simulink library "commanapbnd2"  (Simulink 6.0)
undefined symbols (not defined in the file or in its folder): den, num
libraries: dspsigattribs x26, commanapbnd2 x2, commblksprivate x2, commsynccomp2 x2, dspsrcs4 x1
settings Model: RequirementInfo=9  CovMetricSettings=d  Creator=tdelve  LastModifiedBy=ysong  ExtModeAutoUpdateStatusClock=off

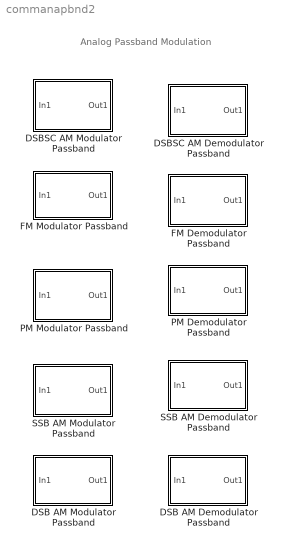
== system commanapbnd2 ==
  note: Analog Passband Modulation
  DSB AM Demodulator Passband : Subsystem  mask(DSB AM Demodulator Passband){Offset=1, Fc=100, Ph=0, num=[4.57 9.14 4.57]*.01, den=[1 -1.3108 .4936], ts=0.001}
      mask prompts: Offset "Offset factor:"; Fc "Carrier frequency (Hz):"; Ph "Initial phase (rad):"; num "Lowpass filter numerator:"; den "Lowpass filter denominator:"; ts "Sample time (s):"
      mask help: Demodulate a double-sideband amplitude modulated signal. The input signal must be a sample-based scalar. The output is a 1-D scalar.
      mask init:
      | if ((length(Ph)~=1) | (length(Offset)~=1) | (length(ts)~=1) | (length(Fc)~=1))error('Mask parameters must be scalar values.');end;
      mask Help: helpview(commbhelp)
      mask Display:
      | plot(0,0,100,100,[5+4.5*[0:.15:10] 50 50 50 50+4.5*[0:10]],[85+10*[sin([0:.15:10]*pi*2+cumsum(sin([0:.15:10]*pi/5))/2)] 85 99 75   10*sin([0:10]*pi/5)+85]);
      | disp('DSB AM')
  DSB AM Modulator Passband : Subsystem  mask(DSB AM Modulator Passband){Offset=1, Fc=100, Ph=0}
      mask prompts: Offset "Input signal offset:"; Fc "Carrier frequency (Hz):"; Ph "Initial phase (rad):"
      mask help: Modulate the input signal using the double-sideband amplitude modulation method. The input signal must be a sample-based scalar. The output is a 1-D scalar.
      mask init:
      | if ((length(Ph)~=1) | (length(Fc)~=1) | (length(Offset)~=1))error('Mask parameters must be scalar values.');end;
      mask Help: helpview(commbhelp)
      mask Display:
      | plot(0,0,100,100,[4.5*[0:10]+5 50 50 50 50+4.5*[0:.15:10]],[10*sin([0:10]*pi/5)+85 85 99 75 85+10*[sin([0:.15:10]*pi*2+cumsum(sin([0:.15:10]*pi/5))/2)]]);
      | disp('DSB AM')
  DSBSC AM Demodulator Passband : Subsystem  mask(DSBSC AM Demodulator Passband){Fc=100, num=[4.57 9.14 4.57]*.01, den=[1 -1.3108 .4936], Ph=pi/2, ts=0.001}
      mask prompts: Fc "Carrier frequency (Hz):"; num "Lowpass filter numerator:"; den "Lowpass filter denominator:"; Ph "Initial phase (rad):"; ts "Sample time (s):"
      mask help: Demodulate a double-sideband suppressed carrier amplitude modulated signal. The input signal must be a sample-based scalar. The output is a 1-D scalar.
      mask init:
      | if ((length(Ph)~=1) | (length(Fc)~=1) | (length(ts)~=1))error('Mask parameters must be scalar values.');end;
      | pi2=pi*2;
      mask Help: helpview(commbhelp)
      mask Display:
      | plot(0,0,100,100,[5+4.5*[0:.15:10] 50 50 50 50+4.5*[0:10]],[85+10*[sin([0:.15:10]*pi*2+cumsum(sin([0:.15:10]*pi/5))/2)] 85 99 75   10*sin([0:10]*pi/5)+85]);
      | disp('DSBSC AM')
  DSBSC AM Modulator Passband : Subsystem  mask(DSBSC AM Modulator Passband){Fc=100, Ph=pi/2}
      mask prompts: Fc "Carrier frequency (Hz):"; Ph "Initial phase (rad):"
      mask help: Modulate the input signal using the double-sideband suppressed carrier amplitude modulation method. The input signal must be a sample-based scalar. The output is a 1-D scalar.
      mask init:
      | if ((length(Ph)~=1) | (length(Fc)~=1))error('Mask parameters must be scalar values.');end;
      | Fc=Fc*2*pi;
      mask Help: helpview(commbhelp)
      mask Display:
      | plot(0,0,100,100,[4.5*[0:10]+5 50 50 50 50+4.5*[0:.15:10]],[10*sin([0:10]*pi/5)+85 85 99 75 85+10*[sin([0:.15:10]*pi*2+cumsum(sin([0:.15:10]*pi/5))/2)]]);
      | disp('DSBSC AM')
  FM Demodulator Passband : Subsystem  mask(FM Demodulator Passband){Fc=100, Ph=0, HzPerVolt=1, num=[4.57 9.14 4.57]*.01, den=[1 -1.3108 .4936], ts=0.001}
      mask prompts: Fc "Carrier frequency (Hz):"; Ph "Initial phase (rad):"; HzPerVolt "Modulation constant (Hertz per volt):"; num "Lowpass filter numerator:"; den "Lowpass filter denominator:"; ts "Sample time (s):"
      mask help: Demodulate a frequency modulated signal using a phase-locked loop. The input signal must be a sample-based scalar. The output is a 1-D scalar.
      mask init:
      | if ((length(Ph)~=1) | (length(HzPerVolt)~=1) | (length(ts)~=1) | (length(Fc)~=1))error('Mask parameters must be scalar values.');end;
      | Ph=Ph+pi/2;
      mask Help: helpview(commbhelp)
      mask Display:
      | plot(0,0,100,100,[5+4.5*[0:.15:10] 50 50 50 50+4.5*[0:10]],[85+10*[sin([0:.15:10]*pi*2+cumsum(sin([0:.15:10]*pi/5))/2)] 85 99 75   10*sin([0:10]*pi/5)+85]);
      | disp('FM')
  FM Modulator Passband : Subsystem  mask(FM Modulator Passband){Fc=100, Ph=0, HzPerV=1, ts=0.001, td=Inf}
      mask prompts: Fc "Carrier frequency (Hz):"; Ph "Initial phase (rad):"; HzPerV "Modulation constant (Hertz per volt):"; ts "Sample time (s):"; td "Symbol interval (s, Use Inf for analog mod);"
      mask help: Modulate the input signal using the frequency modulation method. The input signal must be a sample-based scalar. The output is a 1-D scalar.
      mask init:
      | if ((length(Ph)~=1) | (length(HzPerV)~=1) | (length(ts)~=1) | (length(td)~=1) | (length(Fc)~=1))error('Mask parameters must be scalar values.');end;
      | Kc=HzPerV;pi2=2*pi;if isinf(td),td=realmax;end;
      mask Help: helpview(commbhelp)
      mask Display:
      | plot(0,0,100,100,[4.5*[0:10]+5 50 50 50 50+4.5*[0:.15:10]],[10*sin([0:10]*pi/5)+85 85 99 75 85+10*[sin([0:.15:10]*pi*2+cumsum(sin([0:.15:10]*pi/5))/2)]]);
      | disp('FM')
  PM Demodulator Passband : Subsystem  mask(PM Demodulator Passband){Fc=100, Ph=0, Kc=1, num=[4.57 9.14 4.57]*.01, den=[1 -1.3108 .4936], HzPerVolt=1, ts=0.001}
      mask prompts: Fc "Carrier frequency (Hz):"; Ph "Initial phase (rad):"; Kc "Modulation constant (Radians per volt):"; num "Lowpass filter numerator:"; den "Lowpass filter denominator:"; HzPerVolt "VCO Gain (Hertz per volt):"; ts "Sample time (s):"
      mask help: Demodulate a phase modulated signal using a phase-locked loop. The input signal must be a sample-based scalar. The output is a 1-D scalar.
      mask init:
      | Ph=Ph+pi/2;
      | Kv=2*pi*HzPerVolt;
      mask Help: helpview(commbhelp)
      mask Display:
      | plot(0,0,100,100,[5+4.5*[0:.15:10] 50 50 50 50+4.5*[0:10]],[85+10*[sin([0:.15:10]*pi*2+cumsum(sin([0:.15:10]*pi/5))/2)] 85 99 75   10*sin([0:10]*pi/5)+85]);
      | disp('PM')
  PM Modulator Passband : Subsystem  mask(PM Modulator Passband){Fc=100, Ph=0, Kc=1, td=Inf}
      mask prompts: Fc "Carrier frequency (Hz):"; Ph "Initial phase (rad):"; Kc "Modulation constant (Radians per volt):"; td "Symbol interval (s, Use inf for analog case):"
      mask help: Modulate the input signal using the phase modulation method. The input signal must be a sample-based scalar. The output is a 1-D scalar.
      mask init:
      | if ((length(Ph)~=1) | (length(Kc)~=1) | (length(td)~=1) | (length(Fc)~=1))error('Mask parameters must be scalar values.');end;
      | Fc=Fc*2*pi;if isinf(td),td=realmax;end;
      mask Help: helpview(commbhelp)
      mask Display:
      | plot(0,0,100,100,[4.5*[0:10]+5 50 50 50 50+4.5*[0:.15:10]],[10*sin([0:10]*pi/5)+85 85 99 75 85+10*[sin([0:.15:10]*pi*2+cumsum(sin([0:.15:10]*pi/5))/2)]]);
      | disp('PM')
  SSB AM Demodulator Passband : Subsystem  mask(SSB AM Demodulator Passband){Fc=100, num=[4.57 9.14 4.57]*.01, den=[1 -1.3108 .4936], Ph=0, ts=0.001}
      mask prompts: Fc "Carrier frequency (Hz):"; num "Lowpass filter numerator:"; den "Lowpass filter denominator:"; Ph "Initial phase (rad):"; ts "Sample time (s):"
      mask help: Demodulate a single-sideband amplitude modulated signal. The input signal must be a sample-based scalar. The output is a 1-D scalar.
      mask init:
      | if ((length(Ph)~=1) | (length(Fc)~=1) | (length(ts)~=1))error('Mask parameters must be scalar values.');end;
      | Fc=Fc*2*pi;Pg=Ph+pi/2;
      mask Help: helpview(commbhelp)
      mask Display:
      | plot(0,0,100,100,[5+4.5*[0:.15:10] 50 50 50 50+4.5*[0:10]],[85+10*[sin([0:.15:10]*pi*2+cumsum(sin([0:.15:10]*pi/5))/2)] 85 99 75   10*sin([0:10]*pi/5)+85]);
      | disp('SSB AM')
  SSB AM Modulator Passband : Subsystem  mask(SSB AM Modulator Passband){Fc=100, Ph=0, ban=10, dly=0.01, ts=0.001, sd=upper}
      mask prompts: Fc "Carrier frequency (Hz):"; Ph "Initial phase (rad):"; ban "Bandwidth of the input signal (Hz):"; dly "Time delay for Hilbert transform filter (s):"; ts "Sample time (s):"; sd "Sideband to modulate:"
      mask help: Modulate the input signal using the single-sideband amplitude modulation method with Hilbert transform filter. The input signal must be a sample-based scalar. The output is a 1-D scalar.
      mask init:
      | if ((length(Ph)~=1) | (length(ban)~=1) | (length(ts)~=1) | (length(dly)~=1) | (length(Fc)~=1))error('Mask parameters must be scalar values.');end;
      | if dly/ts<3 error('Time delay is too small compared to the Sample time value');end;
      | if ban>1/ts, ban=1/ts-ts;end;
      | if(dly/ts>1000)
      | error(['The filter coefficients will take too long to compute.'...
      |         'Try reducing the length of the impulse response by increasing the sample time, or decreasing the delay'])
      | else
      | [num,den]=hilbiir(ts,dly,ban);pi2=2*pi;pih=pi/2;
      | k=-1;if lower(sd)=='lower',k=1;end;
      | end;
      mask Help: helpview(commbhelp)
      mask StyleString: edit,edit,edit,edit,edit,popup(Upper|Lower)
      mask Display:
      | plot(0,0,100,100,[4.5*[0:10]+5 50 50 50 50+4.5*[0:.15:10]],[10*sin([0:10]*pi/5)+85 85 99 75 85+10*[sin([0:.15:10]*pi*2+cumsum(sin([0:.15:10]*pi/5))/2)]]);
      | disp('SSB AM')

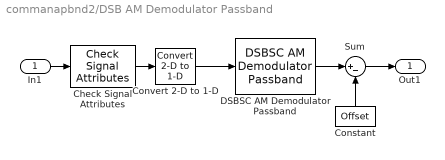
== system commanapbnd2/DSB AM Demodulator Passband ==
  In1 : Inport
  Check Signal Attributes : dspsigattribs/Check Signal Attributes  SigAttribCheckMethod=Does not match attributes exactly  Complexity=Ignore  Frame=Sample-based  DimsCheckMethod=Is...  Dimensions=Scalar (1-D or 2-D)  DatatypeCheckMethod=Ignore  DatatypeGeneral=Boolean  DtypeFloatSpecific=Any floating-point  DtypeFixedSpecific=Any fixed-point  DtypeIntSpecific=Any integer  SampleMode=Ignore
  Constant : Constant  Orientation=up  Value=Offset
  Convert 2-D to 1-D : dspsigattribs/Convert 2-D to 1-D
  DSBSC AM Demodulator Passband : commanapbnd2/DSBSC AM Demodulator Passband  Fc=Fc  num=num  den=den  Ph=Ph  ts=ts
  Sum : Sum  Inputs=|+-  SaturateOnIntegerOverflow=on  InputSameDT=on
  Out1 : Outport
  wires:
  Constant/1 -> Sum/2
  DSBSC AM Demodulator Passband/1 -> Sum/1
  In1/1 -> Check Signal Attributes/1
  Sum/1 -> Out1/1
  Convert 2-D to 1-D/1 -> DSBSC AM Demodulator Passband/1
  Check Signal Attributes/1 -> Convert 2-D to 1-D/1

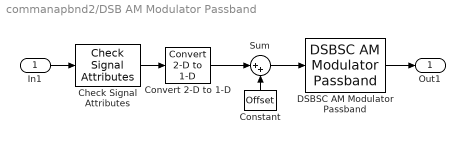
== system commanapbnd2/DSB AM Modulator Passband ==
  In1 : Inport
  Check Signal Attributes : dspsigattribs/Check Signal Attributes  SigAttribCheckMethod=Does not match attributes exactly  Complexity=Ignore  Frame=Sample-based  DimsCheckMethod=Is...  Dimensions=Scalar (1-D or 2-D)  DatatypeCheckMethod=Ignore  DatatypeGeneral=Boolean  DtypeFloatSpecific=Any floating-point  DtypeFixedSpecific=Any fixed-point  DtypeIntSpecific=Any integer  SampleMode=Ignore
  Constant : Constant  Orientation=up  Value=Offset
  Convert 2-D to 1-D : dspsigattribs/Convert 2-D to 1-D
  DSBSC AM Modulator Passband : commanapbnd2/DSBSC AM Modulator Passband  Fc=Fc  Ph=Ph
  Sum : Sum  Inputs=|++  SaturateOnIntegerOverflow=on  InputSameDT=on
  Out1 : Outport
  wires:
  Constant/1 -> Sum/2
  Sum/1 -> DSBSC AM Modulator Passband/1
  In1/1 -> Check Signal Attributes/1
  DSBSC AM Modulator Passband/1 -> Out1/1
  Convert 2-D to 1-D/1 -> Sum/1
  Check Signal Attributes/1 -> Convert 2-D to 1-D/1

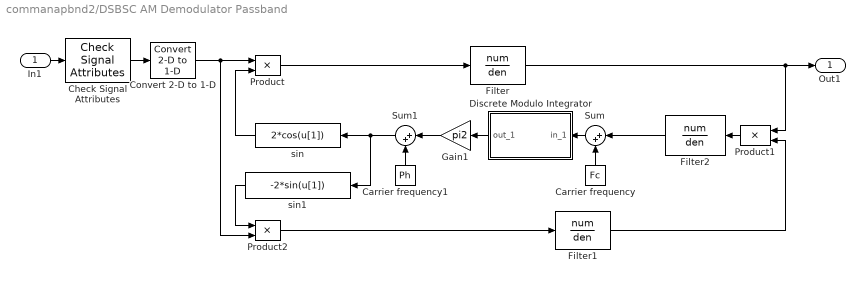
== system commanapbnd2/DSBSC AM Demodulator Passband ==
  In1 : Inport
  Carrier frequency : Constant  Orientation=up  Value=Fc
  Carrier frequency1 : Constant  Orientation=up  Value=Ph
  Check Signal Attributes : dspsigattribs/Check Signal Attributes  SigAttribCheckMethod=Does not match attributes exactly  Complexity=Ignore  Frame=Sample-based  DimsCheckMethod=Is...  Dimensions=Scalar (1-D or 2-D)  DatatypeCheckMethod=Ignore  DatatypeGeneral=Boolean  DtypeFloatSpecific=Any floating-point  DtypeFixedSpecific=Any fixed-point  DtypeIntSpecific=Any integer  SampleMode=Ignore
  Convert 2-D to 1-D : dspsigattribs/Convert 2-D to 1-D
  Discrete Modulo Integrator : Subsystem  Orientation=left  mask(Discrete Modulo Integrator){method=Forward Euler, modu=1, init=0, ts=ts}
      mask prompts: method "Integration method:"; modu "Absolute value bound:"; init "Initial condition:"; ts "Sample time:"
      mask help:
      | Integrate the input signal in discrete time and then uses the Absolute value bound parameter, K, to produce output strictly between -K and K. The block uses the rem function in MATLAB.
      |
      | The input can be either a scalar, a sample-based vector, or a frame-based row vector.  This block processes each vector element independently.
      mask init:
      | commblkdmodint(gcb);
      settings: ErrorFcn=commblkdmint
      mask Help: helpview(commbhelp)
      mask StyleString: popup(Forward Euler|Backward Euler|Trapezoidal),edit,edit,edit
      mask Display: disp('Discrete\nModulo\nIntegrator')
  Filter : DiscreteFilter  Numerator=num  Denominator=den  SampleTime=ts
  Filter1 : DiscreteFilter  Numerator=num  Denominator=den  SampleTime=ts
  Filter2 : DiscreteFilter  Orientation=left  Numerator=num  Denominator=den  SampleTime=ts
  Gain1 : Gain  Orientation=left  Gain=pi2  SaturateOnIntegerOverflow=on
  Product : Product  SaturateOnIntegerOverflow=on  InputSameDT=on
  Product1 : Product  Orientation=left  SaturateOnIntegerOverflow=on  InputSameDT=on
  Product2 : Product  SaturateOnIntegerOverflow=on  InputSameDT=on
  Sum : Sum  Orientation=left  Inputs=|++  SaturateOnIntegerOverflow=on  InputSameDT=on
  Sum1 : Sum  Orientation=left  Inputs=|++  SaturateOnIntegerOverflow=on  InputSameDT=on
  sin : Fcn  Orientation=left  Expr=2*cos(u[1])
  sin1 : Fcn  Orientation=left  Expr=-2*sin(u[1])
  Out1 : Outport
  wires:
  Sum1/1 -> sin/1, sin1/1
  Filter2/1 -> Sum/1
  Product/1 -> Filter/1
  sin/1 -> Product/2
  Carrier frequency/1 -> Sum/2
  Sum/1 -> Discrete Modulo Integrator/1(in_1)
  Product1/1 -> Filter2/1
  sin1/1 -> Product2/1
  In1/1 -> Check Signal Attributes/1
  Product2/1 -> Filter1/1
  Filter1/1 -> Product1/2
  Discrete Modulo Integrator/1(out_1) -> Gain1/1
  Gain1/1 -> Sum1/1
  Carrier frequency1/1 -> Sum1/2
  Filter/1 -> Product1/1, Out1/1
  Convert 2-D to 1-D/1 -> Product/1, Product2/2
  Check Signal Attributes/1 -> Convert 2-D to 1-D/1

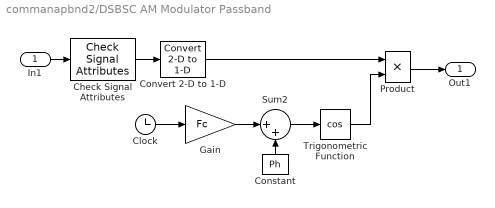
== system commanapbnd2/DSBSC AM Modulator Passband ==
  In1 : Inport
  Check Signal Attributes : dspsigattribs/Check Signal Attributes  SigAttribCheckMethod=Does not match attributes exactly  Complexity=Ignore  Frame=Sample-based  DimsCheckMethod=Is...  Dimensions=Scalar (1-D or 2-D)  DatatypeCheckMethod=Ignore  DatatypeGeneral=Boolean  DtypeFloatSpecific=Any floating-point  DtypeFixedSpecific=Any fixed-point  DtypeIntSpecific=Any integer  SampleMode=Ignore
  Clock : Clock
      settings: Decimation=10
  Constant : Constant  Orientation=up  Value=Ph
  Convert 2-D to 1-D : dspsigattribs/Convert 2-D to 1-D
  Gain : Gain  Gain=Fc  SaturateOnIntegerOverflow=on
  Product : Product  SaturateOnIntegerOverflow=on  InputSameDT=on
  Sum2 : Sum  Inputs=|++  SaturateOnIntegerOverflow=on  InputSameDT=on
  Trigonometric Function : Trigonometry  Operator=cos
  Out1 : Outport
  wires:
  Trigonometric Function/1 -> Product/2
  In1/1 -> Check Signal Attributes/1
  Clock/1 -> Gain/1
  Gain/1 -> Sum2/1
  Constant/1 -> Sum2/2
  Sum2/1 -> Trigonometric Function/1
  Product/1 -> Out1/1
  Convert 2-D to 1-D/1 -> Product/1
  Check Signal Attributes/1 -> Convert 2-D to 1-D/1

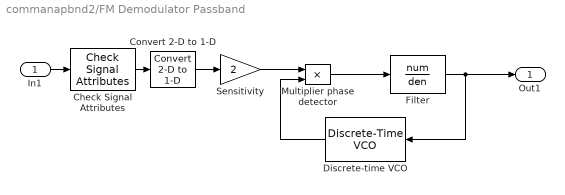
== system commanapbnd2/FM Demodulator Passband ==
  In1 : Inport
  Check Signal Attributes : dspsigattribs/Check Signal Attributes  SigAttribCheckMethod=Does not match attributes exactly  Complexity=Ignore  Frame=Sample-based  DimsCheckMethod=Is...  Dimensions=Scalar (1-D or 2-D)  DatatypeCheckMethod=Ignore  DatatypeGeneral=Boolean  DtypeFloatSpecific=Any floating-point  DtypeFixedSpecific=Any fixed-point  DtypeIntSpecific=Any integer  SampleMode=Ignore
  Convert 2-D to 1-D : dspsigattribs/Convert 2-D to 1-D
  Discrete-time VCO : commsynccomp2/Discrete-Time VCO  Orientation=left  Ac=1  Fc=Fc  Kc=HzPerVolt  Ph=Ph  ts=ts
  Filter : DiscreteFilter  Numerator=num  Denominator=den  SampleTime=ts
  Multiplier phase detector : Product  SaturateOnIntegerOverflow=on  InputSameDT=on
  Sensitivity : Gain  Gain=2  SaturateOnIntegerOverflow=on
  Out1 : Outport
  wires:
  Discrete-time VCO/1 -> Multiplier phase detector/2
  Multiplier phase detector/1 -> Filter/1
  Filter/1 -> Discrete-time VCO/1, Out1/1
  In1/1 -> Check Signal Attributes/1
  Sensitivity/1 -> Multiplier phase detector/1
  Convert 2-D to 1-D/1 -> Sensitivity/1
  Check Signal Attributes/1 -> Convert 2-D to 1-D/1

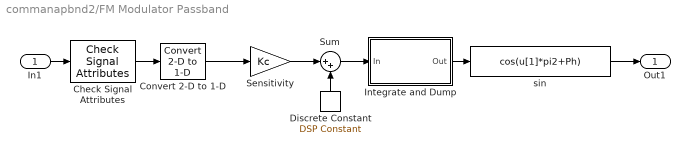
== system commanapbnd2/FM Modulator Passband ==
  In1 : Inport
  Check Signal Attributes : dspsigattribs/Check Signal Attributes  SigAttribCheckMethod=Does not match attributes exactly  Complexity=Ignore  Frame=Sample-based  DimsCheckMethod=Is...  Dimensions=Scalar (1-D or 2-D)  DatatypeCheckMethod=Ignore  DatatypeGeneral=Boolean  DtypeFloatSpecific=Any floating-point  DtypeFixedSpecific=Any fixed-point  DtypeIntSpecific=Any integer  SampleMode=Ignore
  Convert 2-D to 1-D : dspsigattribs/Convert 2-D to 1-D
  Discrete Constant : dspsrcs4/DSP Constant  Orientation=up  Value=Fc  SampleMode=Discrete  discreteOutput=Sample-based (interpret vectors as 1-D)  continuousOutput=Sample-based  sampTime=ts  framePeriod=ts  dataType=Inherit from 'Constant value'  wordLen=16  udDataType=sfix(16)  fracBitsMode=Best precision  numFracBits=15  InterpretAs1D=on  Ts=ts  FramebasedOutput=off
  Integrate and Dump : Subsystem  mask(Integrate and Dump){limit=Inf/2, td=td, ts=ts}
      mask prompts: limit "Absolute value bound:"; td "Integration period (s):"; ts "Sample time:"
      mask help:
      | Integrate the input signal in discrete time over the Integration period and then reduce modulo the Absolute value bound parameter. The integrator resets its internal state before integrating the next period.
      |
      | The input can be either a scalar, a sample-based vector, or a frame-based row vector.  This block processes each vector element independently.
      mask init:
      | limit(find(isinf(limit))) = realmax;
      | td(find(isinf(td))) = realmax;
      | 
      | if(~isempty(ts))
      |    if(length(ts) ~= 1)
      |       error('Sample time parameter must be a real scalar.');
      |    end;
      | end;
      settings: ErrorFcn=commblkintdmp
      mask Help: helpview(commbhelp)
      mask Display: disp('Integrate\nand Dump')
  Sensitivity : Gain  Gain=Kc  SaturateOnIntegerOverflow=on
  Sum : Sum  Inputs=|++  SaturateOnIntegerOverflow=on  InputSameDT=on
  sin : Fcn  Expr=cos(u[1]*pi2+Ph)
  Out1 : Outport
  wires:
  Integrate and Dump/1(Out) -> sin/1
  Sum/1 -> Integrate and Dump/1(In)
  In1/1 -> Check Signal Attributes/1
  Sensitivity/1 -> Sum/1
  sin/1 -> Out1/1
  Convert 2-D to 1-D/1 -> Sensitivity/1
  Check Signal Attributes/1 -> Convert 2-D to 1-D/1
  Discrete Constant/1 -> Sum/2

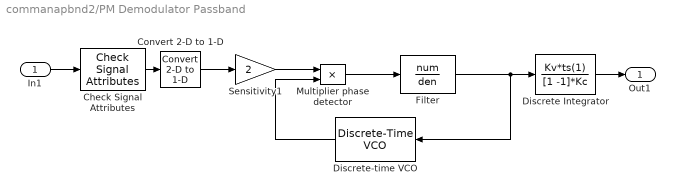
== system commanapbnd2/PM Demodulator Passband ==
  In1 : Inport
  Check Signal Attributes : dspsigattribs/Check Signal Attributes  SigAttribCheckMethod=Does not match attributes exactly  Complexity=Ignore  Frame=Sample-based  DimsCheckMethod=Is...  Dimensions=Scalar (1-D or 2-D)  DatatypeCheckMethod=Ignore  DatatypeGeneral=Boolean  DtypeFloatSpecific=Any floating-point  DtypeFixedSpecific=Any fixed-point  DtypeIntSpecific=Any integer  SampleMode=Ignore
  Convert 2-D to 1-D : dspsigattribs/Convert 2-D to 1-D
  Discrete Integrator : DiscreteFilter  Numerator=Kv*ts(1)  Denominator=[1 -1]*Kc  SampleTime=ts
  Discrete-time VCO : commsynccomp2/Discrete-Time VCO  Orientation=left  Ac=1  Fc=Fc  Kc=HzPerVolt  Ph=Ph  ts=ts
  Filter : DiscreteFilter  Numerator=num  Denominator=den  SampleTime=ts
  Multiplier phase detector : Product  SaturateOnIntegerOverflow=on  InputSameDT=on
  Sensitivity1 : Gain  Gain=2  SaturateOnIntegerOverflow=on
  Out1 : Outport  InitialOutput=0
  wires:
  Discrete-time VCO/1 -> Multiplier phase detector/2
  Filter/1 -> Discrete-time VCO/1, Discrete Integrator/1
  Multiplier phase detector/1 -> Filter/1
  In1/1 -> Check Signal Attributes/1
  Sensitivity1/1 -> Multiplier phase detector/1
  Discrete Integrator/1 -> Out1/1
  Convert 2-D to 1-D/1 -> Sensitivity1/1
  Check Signal Attributes/1 -> Convert 2-D to 1-D/1

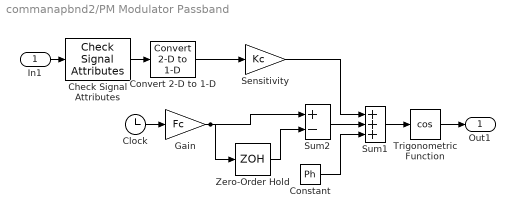
== system commanapbnd2/PM Modulator Passband ==
  In1 : Inport
  Check Signal Attributes : dspsigattribs/Check Signal Attributes  SigAttribCheckMethod=Does not match attributes exactly  Complexity=Ignore  Frame=Sample-based  DimsCheckMethod=Is...  Dimensions=Scalar (1-D or 2-D)  DatatypeCheckMethod=Ignore  DatatypeGeneral=Boolean  DtypeFloatSpecific=Any floating-point  DtypeFixedSpecific=Any fixed-point  DtypeIntSpecific=Any integer  SampleMode=Ignore
  Clock : Clock
      settings: Decimation=10
  Constant : Constant  Value=Ph
  Convert 2-D to 1-D : dspsigattribs/Convert 2-D to 1-D
  Gain : Gain  Gain=Fc  SaturateOnIntegerOverflow=on
  Sensitivity : Gain  Gain=Kc  SaturateOnIntegerOverflow=on
  Sum1 : Sum  Inputs=+++  SaturateOnIntegerOverflow=on  InputSameDT=on
  Sum2 : Sum  Inputs=+-  SaturateOnIntegerOverflow=on  InputSameDT=on
  Trigonometric Function : Trigonometry  Operator=cos
  Zero-Order Hold : ZeroOrderHold  SampleTime=td
  Out1 : Outport
  wires:
  Constant/1 -> Sum1/3
  Sum1/1 -> Trigonometric Function/1
  Clock/1 -> Gain/1
  Sum2/1 -> Sum1/2
  Zero-Order Hold/1 -> Sum2/2
  Gain/1 -> Sum2/1, Zero-Order Hold/1
  In1/1 -> Check Signal Attributes/1
  Sensitivity/1 -> Sum1/1
  Trigonometric Function/1 -> Out1/1
  Convert 2-D to 1-D/1 -> Sensitivity/1
  Check Signal Attributes/1 -> Convert 2-D to 1-D/1

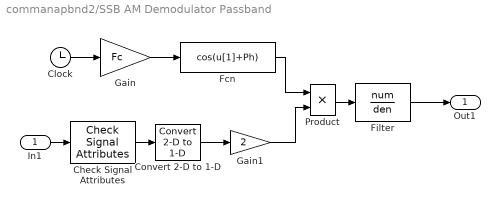
== system commanapbnd2/SSB AM Demodulator Passband ==
  In1 : Inport
  Check Signal Attributes : dspsigattribs/Check Signal Attributes  SigAttribCheckMethod=Does not match attributes exactly  Complexity=Ignore  Frame=Sample-based  DimsCheckMethod=Is...  Dimensions=Scalar (1-D or 2-D)  DatatypeCheckMethod=Ignore  DatatypeGeneral=Boolean  DtypeFloatSpecific=Any floating-point  DtypeFixedSpecific=Any fixed-point  DtypeIntSpecific=Any integer  SampleMode=Ignore
  Clock : Clock
      settings: Decimation=10
  Convert 2-D to 1-D : dspsigattribs/Convert 2-D to 1-D
  Fcn : Fcn  Expr=cos(u[1]+Ph)
  Filter : DiscreteFilter  Numerator=num  Denominator=den  SampleTime=ts
  Gain : Gain  Gain=Fc  SaturateOnIntegerOverflow=on
  Gain1 : Gain  Gain=2  SaturateOnIntegerOverflow=on
  Product : Product  SaturateOnIntegerOverflow=on  InputSameDT=on
  Out1 : Outport
  wires:
  Clock/1 -> Gain/1
  Product/1 -> Filter/1
  Fcn/1 -> Product/1
  Gain1/1 -> Product/2
  Gain/1 -> Fcn/1
  Filter/1 -> Out1/1
  Convert 2-D to 1-D/1 -> Gain1/1
  Check Signal Attributes/1 -> Convert 2-D to 1-D/1
  In1/1 -> Check Signal Attributes/1

== system commanapbnd2/SSB AM Modulator Passband ==
  In1 : Inport
  Check Signal Attributes : dspsigattribs/Check Signal Attributes  SigAttribCheckMethod=Does not match attributes exactly  Complexity=Ignore  Frame=Sample-based  DimsCheckMethod=Is...  Dimensions=Scalar (1-D or 2-D)  DatatypeCheckMethod=Ignore  DatatypeGeneral=Boolean  DtypeFloatSpecific=Any floating-point  DtypeFixedSpecific=Any fixed-point  DtypeIntSpecific=Any integer  SampleMode=Ignore
  Convert 2-D to 1-D : dspsigattribs/Convert 2-D to 1-D
  Filter : DiscreteFilter  Numerator=num  Denominator=den  SampleTime=ts
  Gain : Gain  Gain=k  SaturateOnIntegerOverflow=on
  QAM passband : Subsystem  mask(QAM Passband){Fc=Fc, Ph=Ph}
      mask prompts: Fc "Carrier frequency (Hz):"; Ph "Initial phase (rad):"
      mask help: Modulate the in-phase signal from first input port and quadrature signal from the second port using QAM.
      mask init:
      | Fc=Fc*2*pi;
      mask Help: helpview(commbhelp)
      mask Display:
      | plot(0,0,100,100,[4.5*[0:10]+5 50 50 50 50+4.5*[0:.3:10]],[10*sin([0:10]*pi/5)+85 85 99 75 85+10*[sin([0:.3:10]*pi/5).*sin([0:.3:10]*pi*2)]]);
      | disp('\nPassband\nQAM')
  Out1 : Outport
  wires:
  In1/1 -> Check Signal Attributes/1
  Filter/1 -> Gain/1
  Gain/1 -> QAM passband/2(in_2)
  QAM passband/1(out_1) -> Out1/1
  Convert 2-D to 1-D/1 -> QAM passband/1(in_1), Filter/1
  Check Signal Attributes/1 -> Convert 2-D to 1-D/1

== system commanapbnd2/DSBSC AM Demodulator Passband/Discrete Modulo Integrator ==
  in_1 : Inport
  Discrete Modulo Integrator : Subsystem
  "Exclude Frame-based Input " : dspsigattribs/Check Signal Attributes  SigAttribCheckMethod=Matches attributes exactly  Complexity=Ignore  Frame=Frame-based  DimsCheckMethod=Is not...  Dimensions=Row vector (2-D) or scalar  DatatypeCheckMethod=Ignore  DatatypeGeneral=Boolean  DtypeFloatSpecific=Any floating-point  DtypeFixedSpecific=Any fixed-point  DtypeIntSpecific=Any integer  SampleMode=Ignore
  Exclude Full Matrix : dspsigattribs/Check Signal Attributes  SigAttribCheckMethod=Matches attributes exactly  Complexity=Ignore  Frame=Ignore  DimsCheckMethod=Is...  Dimensions=Full matrix (2-D)  DatatypeCheckMethod=Ignore  DatatypeGeneral=Boolean  DtypeFloatSpecific=Any floating-point  DtypeFixedSpecific=Any fixed-point  DtypeIntSpecific=Any integer  SampleMode=Ignore
  Frame Status Conversion : dspsigattribs/Frame Status Conversion  growRefPort=off  outframe=Sample-based
  Inherit Shape : commblksprivate/Inherit Shape
  out_1 : Outport  InitialOutput=0
  wires:
  Discrete Modulo Integrator/1(Out1) -> Inherit Shape/1
  Frame Status Conversion/1 -> Discrete Modulo Integrator/1(In1)
  "Exclude Frame-based Input "/1 -> Frame Status Conversion/1
  Exclude Full Matrix/1 -> "Exclude Frame-based Input "/1
  Inherit Shape/1 -> out_1/1
  in_1/1 -> Inherit Shape/2, Exclude Full Matrix/1

== system commanapbnd2/FM Modulator Passband/Integrate and Dump ==
  In : Inport
  "Exclude Frame-based Input " : dspsigattribs/Check Signal Attributes  SigAttribCheckMethod=Matches attributes exactly  Complexity=Ignore  Frame=Frame-based  DimsCheckMethod=Is not...  Dimensions=Row vector (2-D) or scalar  DatatypeCheckMethod=Ignore  DatatypeGeneral=Boolean  DtypeFloatSpecific=Any floating-point  DtypeFixedSpecific=Any fixed-point  DtypeIntSpecific=Any integer  SampleMode=Ignore
  Exclude Full Matrix : dspsigattribs/Check Signal Attributes  SigAttribCheckMethod=Matches attributes exactly  Complexity=Ignore  Frame=Ignore  DimsCheckMethod=Is...  Dimensions=Full matrix (2-D)  DatatypeCheckMethod=Ignore  DatatypeGeneral=Boolean  DtypeFloatSpecific=Any floating-point  DtypeFixedSpecific=Any fixed-point  DtypeIntSpecific=Any integer  SampleMode=Ignore
  Frame Status Conversion : dspsigattribs/Frame Status Conversion  growRefPort=off  outframe=Sample-based
  Inherit Shape : commblksprivate/Inherit Shape
  Scheduled reset-int : S-Function  FunctionName=schdint  Parameters=td, ts, limit
  Out : Outport  InitialOutput=0
  wires:
  Exclude Full Matrix/1 -> "Exclude Frame-based Input "/1
  "Exclude Frame-based Input "/1 -> Frame Status Conversion/1
  Frame Status Conversion/1 -> Scheduled reset-int/1
  Inherit Shape/1 -> Out/1
  Scheduled reset-int/1 -> Inherit Shape/1
  In/1 -> Inherit Shape/2, Exclude Full Matrix/1

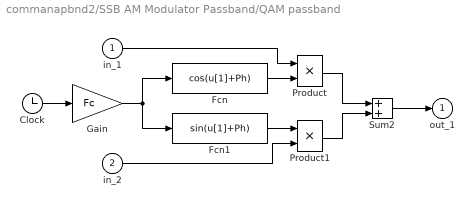
== system commanapbnd2/SSB AM Modulator Passband/QAM passband ==
  in_1 : Inport
  in_2 : Inport  Port=2
  Clock : Clock
      settings: Decimation=10
  Fcn : Fcn  Expr=cos(u[1]+Ph)
  Fcn1 : Fcn  Expr=sin(u[1]+Ph)
  Gain : Gain  Gain=Fc  SaturateOnIntegerOverflow=on
  Product : Product  SaturateOnIntegerOverflow=on  InputSameDT=on
  Product1 : Product  SaturateOnIntegerOverflow=on  InputSameDT=on
  Sum2 : Sum  SaturateOnIntegerOverflow=on  InputSameDT=on
  out_1 : Outport  InitialOutput=0
  wires:
  Sum2/1 -> out_1/1
  Fcn/1 -> Product/2
  in_1/1 -> Product/1
  Fcn1/1 -> Product1/1
  in_2/1 -> Product1/2
  Product/1 -> Sum2/1
  Product1/1 -> Sum2/2
  Clock/1 -> Gain/1
  Gain/1 -> Fcn1/1, Fcn/1

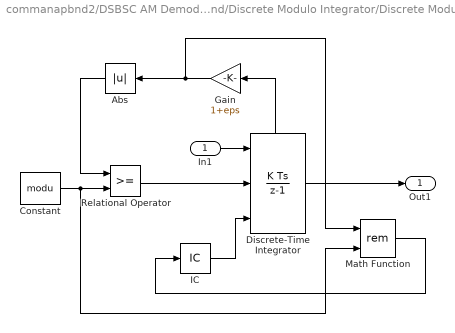
== system commanapbnd2/DSBSC AM Demodulator Passband/Discrete Modulo Integrator/Discrete Modulo Integrator ==
  In1 : Inport
  Abs : Abs  Orientation=left  SaturateOnIntegerOverflow=on
  Constant : Constant  Value=modu
  Discrete-Time Integrator : DiscreteIntegrator  ExternalReset=rising  InitialConditionSource=external  UpperSaturationLimit=2*modu  LowerSaturationLimit=-2*modu  ShowStatePort=on  SampleTime=ts
  Gain : Gain  Orientation=left  Gain=1+eps  SaturateOnIntegerOverflow=on
  IC : InitialCondition  Value=init
  Math Function : Math  Operator=rem  SaturateOnIntegerOverflow=on
  Relational Operator : RelationalOperator  InputSameDT=on
  Out1 : Outport
  wires:
  Gain/1 -> Math Function/1, Abs/1
  In1/1 -> Discrete-Time Integrator/1
  Constant/1 -> Relational Operator/2, Math Function/2
  Abs/1 -> Relational Operator/1
  Discrete-Time Integrator/State -> Gain/1
  Relational Operator/1 -> Discrete-Time Integrator/2
  Math Function/1 -> IC/1
  Discrete-Time Integrator/1 -> Out1/1
  IC/1 -> Discrete-Time Integrator/3
